simulink model "HeadingMode"  (R2012b)
settings: configuration reference "configSetObj_autopilot" (kept outside this file)
undefined symbols (not defined in the file or in its folder): hdgGain
settings Model: Creator=ssauvage  LastModifiedBy=ssauvage

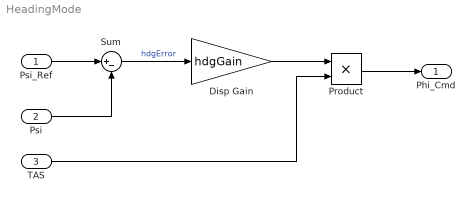
== system HeadingMode ==
  Psi_Ref : Inport  RequirementInfo={} %GIDa_62cbcee6_e6c6_4e91_9e20_02dc12332ed2  OutDataTypeStr=double  PortDimensions=1  SampleTime=1/40  Interpolate=off
  Psi : Inport  RequirementInfo={} %GIDa_c894a55b_5c64_46b5_949c_1d9c7ccbe81c  Port=2  OutDataTypeStr=double  PortDimensions=1  SampleTime=1/40  Interpolate=off
  TAS : Inport  RequirementInfo={} %GIDa_5fc90bd0_1b63_4edb_acd4_8a2db71e1a1b  Port=3  OutDataTypeStr=double  PortDimensions=1  SampleTime=1/40  Interpolate=off
  Disp Gain : Gain  RequirementInfo={} %GIDa_c2e90797_5fde_4195_bffb_596e7c6bc0f3  Gain=hdgGain
  Product : Product  RequirementInfo={} %GIDa_e85e279a_5745_4bcb_b868_820cb71ea6f4  RndMeth=Zero
  Sum : Sum  RequirementInfo={} %GIDa_4531b595_91b7_466d_a25d_f410a52ca8ce  Inputs=|+-
  Phi_Cmd : Outport  RequirementInfo={} %GIDa_26a99a15_245c_4ee5_96ef_7d83a76f5706  OutDataTypeStr=double  PortDimensions=1  SampleTime=1/40
  wires:
  Product/1 -> Phi_Cmd/1
  Disp Gain/1 -> Product/1
  Sum/1 -> Disp Gain/1  "hdgError"
  Psi/1 -> Sum/2
  Psi_Ref/1 -> Sum/1
  TAS/1 -> Product/2
